simulink model "modelo8_simulink_controle_integral"  (R2023b)
settings: Solver=VariableStepAuto  StartTime=0.0  StopTime=15  RelTol=1e-3
undefined symbols (not defined in the file or in its folder): Ar, Br, C_psi, Cr, Cref, F_psi, Ki, Kx
settings Model: Creator=Talles  LastModifiedBy=Talles
settings DataIOCC: Refine=10

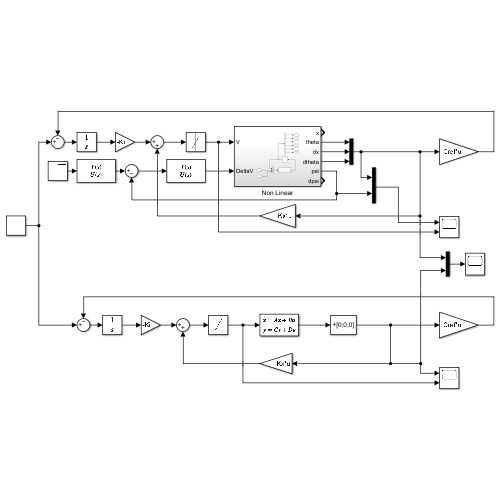
[thumbnail: Simulink's stored preview of the top-level diagram]
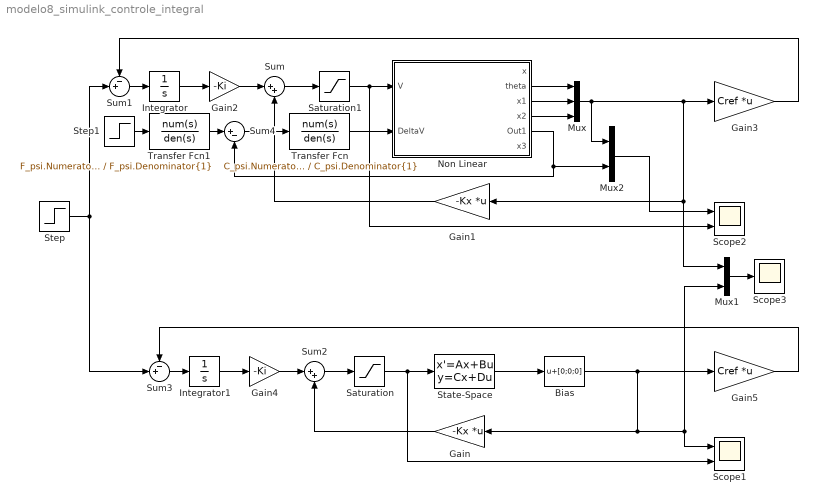
== system modelo8_simulink_controle_integral ==
  Bias : Bias  Bias=[0;0;0]  SaturateOnIntegerOverflow=off
  Gain : Gain  Gain=-Kx  Multiplication=Matrix(K*u)
  Gain1 : Gain  Gain=-Kx  Multiplication=Matrix(K*u)
  Gain2 : Gain  Gain=-Ki
  Gain3 : Gain  Gain=Cref  Multiplication=Matrix(K*u)
  Gain4 : Gain  Gain=-Ki
  Gain5 : Gain  Gain=Cref  Multiplication=Matrix(K*u)
  Integrator : Integrator
  Integrator1 : Integrator
  Mux : Mux  Inputs=3
  Mux1 : Mux  Inputs=2
  Mux2 : Mux  Inputs=2
  Non Linear : Subsystem
  Saturation : Saturate  UpperLimit=7.4  LowerLimit=-7.4
  Saturation1 : Saturate  UpperLimit=7.4  LowerLimit=-7.4
  Scope1 : Scope  NumInputPorts=2
  Scope2 : Scope  NumInputPorts=2
  Scope3 : Scope
  State-Space : StateSpace  A=Ar  B=Br  C=Cr  D=zeros(3,1)  InitialCondition=zeros(3,1)
  Step : Step  Time=5  After=0.5  SampleTime=0
  Step1 : Step  Time=10  After=pi/2  SampleTime=0
  Sum : Sum  Inputs=|++
  Sum1 : Sum  Inputs=-+|
  Sum2 : Sum  Inputs=|++
  Sum3 : Sum  Inputs=-+|
  Sum4 : Sum  Inputs=|+-
  Transfer Fcn : TransferFcn  Numerator=C_psi.Numerator{1}  Denominator=C_psi.Denominator{1}
  Transfer Fcn1 : TransferFcn  Numerator=F_psi.Numerator{1}  Denominator=F_psi.Denominator{1}
  wires:
  State-Space/1 -> Bias/1
  Bias/1 -> Mux1/2, Scope1/1, Gain/1, Gain5/1
  Saturation/1 -> Scope1/2, State-Space/1
  Non Linear/2(theta) -> Mux/1
  Non Linear/3(x1) -> Mux/2
  Gain1/1 -> Sum/2
  Saturation1/1 -> Non Linear/1(V), Scope2/2
  Non Linear/4(x2) -> Mux/3
  Mux1/1 -> Scope3/1
  Mux/1 -> Mux2/1, Gain3/1, Mux1/1, Gain1/1
  Sum/1 -> Saturation1/1
  Integrator/1 -> Gain2/1
  Gain2/1 -> Sum/1
  Gain3/1 -> Sum1/1
  Sum1/1 -> Integrator/1
  Step/1 -> Sum3/2, Sum1/2
  Sum3/1 -> Integrator1/1
  Gain4/1 -> Sum2/1
  Integrator1/1 -> Gain4/1
  Sum2/1 -> Saturation/1
  Gain/1 -> Sum2/2
  Gain5/1 -> Sum3/1
  Transfer Fcn/1 -> Non Linear/2(DeltaV)
  Sum4/1 -> Transfer Fcn/1
  Non Linear/5(Out1) -> Mux2/2, Sum4/2
  Mux2/1 -> Scope2/1
  Transfer Fcn1/1 -> Sum4/1
  Step1/1 -> Transfer Fcn1/1

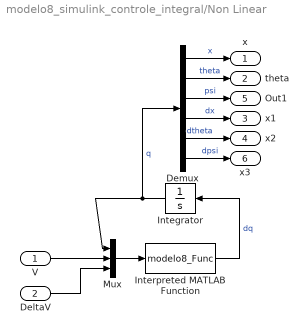
== system modelo8_simulink_controle_integral/Non Linear ==
  V : Inport
  DeltaV : Inport  Port=2
  Demux : Demux  Outputs=6
  Integrator : Integrator  InitialCondition=[0;0;0;0;0;0]
  Interpreted MATLAB Function : MATLABFcn  MATLABFcn=modelo8_Func  OutputDimensions=6  OutputSignalType=real
  Mux : Mux  Inputs=3
  x : Outport
  theta : Outport  Port=2
  x1 : Outport  Port=3
  x2 : Outport  Port=4
  Out1 : Outport  Port=5
  x3 : Outport  Port=6
  wires:
  Interpreted MATLAB Function/1 -> Integrator/1  "dq"
  Integrator/1 -> Demux/1, Mux/1  "q"
  Demux/3 -> Out1/1  "psi"
  Mux/1 -> Interpreted MATLAB Function/1
  Demux/1 -> x/1  "x"
  Demux/2 -> theta/1  "theta"
  V/1 -> Mux/2
  Demux/4 -> x1/1  "dx"
  Demux/5 -> x2/1  "dtheta"
  Demux/6 -> x3/1  "dpsi"
  DeltaV/1 -> Mux/3
